simulink model "SDV_HIL"  (R2025a)
settings: Solver=VariableStepAuto  StartTime=0.0  StopTime=9999  FixedStep=0.001  RelTol=1e-3
undefined symbols (not defined in the file): Breakpoints_Fz, Cij, dspblkCoreblockFVToolHelper, eta, Fx_total_max, g, gcbh, Iz, lambda, lf, lr, mu, phi, R_eff, Tmax, xi
libraries: simulink_extras x30, slrealtimeiplib x17, slpidlib x16, simulink x10, SignalEditorBlockLib x6, dspstat3 x5, Solver_SF x3, sl3dlib x3
(part 4 of 5)

== system SDV_HIL/Draft1/UDP Transmit PC -> VCU1/Subsystem/Torque Vectoring/Speed Control ==
  Vx_des : Inport
  Vx : Inport  Port=2
  Display : Display  Commented=on
  MATLAB Function : MATLAB Function  TreatAsAtomicUnit=on
  Mux : Mux  Inputs=2
  PID Controller4 : slpidlib/PID Controller  Controller=PID  Form=Parallel  TimeDomain=Discrete-time  UseExternalTs=off  SampleTime=-1  IntegratorMethod=Forward Euler  FilterMethod=Forward Euler  ControllerParametersSource=internal  P=1500  I=2  UseKiTs=off  D=30  UseExternalDerivativeSource=off  N=100  UseFilter=on  TunerSelectOption=Transfer Function Based (PID Tuner App)  InitialConditionSource=internal  InitialConditionForIntegrator=0  InitialConditionForFilter=0  DifferentiatorICPrevScaledInput=0  ExternalReset=none  TrackingMode=off  Kt=1  LimitOutput=off  SatLimitsSource=internal  UpperSaturationLimit=inf  LowerSaturationLimit=-inf  LinearizeAsGain=on  AntiWindupMode=none  Kb=1  LimitIntegrator=off  UpperIntegratorSaturationLimit=inf  LowerIntegratorSaturationLimit=-inf  POutMin=[]  POutMax=[]  IOutMin=[]  IOutMax=[]  DOutMin=[]  DOutMax=[]  NOutMin=[]  NOutMax=[]  SumOutMin=[]  SumOutMax=[]  SaturationOutMin=[]  SaturationOutMax=[]  PParamMin=[]  PParamMax=[]  IParamMin=[]  IParamMax=[]  DParamMin=[]  DParamMax=[]  NParamMin=[]  NParamMax=[]  KbParamMin=[]  KbParamMax=[]  KtParamMin=[]  KtParamMax=[]  KbOutMin=[]  KbOutMax=[]  KtOutMin=[]  KtOutMax=[]  IntegratorOutMin=[]  IntegratorOutMax=[]  FilterOutMin=[]  FilterOutMax=[]  SumI1OutMin=[]  SumI1OutMax=[]  SumI2OutMin=[]  SumI2OutMax=[]  SumI3OutMin=[]  SumI3OutMax=[]  SumI4OutMin=[]  SumI4OutMax=[]  SumDOutMin=[]  SumDOutMax=[]  DifferentiatorOutMin=[]  DifferentiatorOutMax=[]  FilterDiffOutCoefMin=[]  FilterDiffOutCoefMax=[]  ReciprocalOutMin=[]  ReciprocalOutMax=[]  SumDenOutMin=[]  SumDenOutMax=[]  SumNumOutMin=[]  SumNumOutMax=[]  DivideOutMin=[]  DivideOutMax=[]  UdiffTsProdOutMin=[]  UdiffTsProdOutMax=[]  NTsProdOutMin=[]  NTsProdOutMax=[]  UintegralTsProdOutMin=[]  UintegralTsProdOutMax=[]  UngainTsProdOutMin=[]  UngainTsProdOutMax=[]  ClampingZeroOutDataTypeStr=Inherit: Inherit via back propagation  ClampingZeroOutMin=[]  ClampingZeroOutMax=[]  FilterDenConstantOutDataTypeStr=Inherit: Inherit via back propagation  FilterDenConstantOutMin=[]  FilterDenConstantOutMax=[]  PCopyOutDataTypeStr=Inherit: Inherit via back propagation  PCopyOutMin=[]  PCopyOutMax=[]  NCopyOutDataTypeStr=Inherit: Inherit via back propagation  NCopyOutMin=[]  NCopyOutMax=[]  IntegratorContinuousStateAttributes=''  IntegratorStateMustResolveToSignalObject=off  IntegratorRTWStateStorageClass=Auto  FilterContinuousStateAttributes=''  FilterStateMustResolveToSignalObject=off  FilterRTWStateStorageClass=Auto  ParallelPVariant=InternalParameters  IdealPVariant=Disabled  IVariant=InternalParameters  DVariant=InternalParameters  IntegratorVariant=Discrete  SatVariant=Disabled  AWVariant=Passthrough  PCopyVariant=Disabled  TRVariant=Disabled  FdbkBlocksVariant=Forward  IdealPFdbkVariant=Disabled  SatFdbkVariant=Disabled  DerivativeFilterVariant=ForwardEulerFilter  NVariant=InternalParameters  NCopyVariant=Disabled  FilterICVariant=InternalICsFilter  IntegratorICVariant=InternalICs  ExternalResetVariant=Disabled  TRSumVariant=Passthrough  SumFdbkVariant=Disabled  SumVariant=Sum_PID  TsampFilterVariant=InternalTs  TsampNgainVariant=Passthrough  TsampIntegralVariant=Disabled_SignalSpec  ExternalSaturationOutDataTypeStr=Inherit: Same as second input  DerivativeSourceVariant=ErrorSignal  PreIntVariant=InternalPreInt
  Saturation : Saturate  UpperLimit=Fx_total_max  LowerLimit=0
  Scope : Scope  Commented=on  NumInputPorts=2
      settings: ActiveDisplayYMinimum=-2.88760628149626  ActiveDisplayYMaximum=25.98790920244803  DataLoggingVariableName=ScopeData38
  Scope1 : Scope  Commented=on
      settings: ActiveDisplayYMinimum=-1  ActiveDisplayYMaximum=1  DataLoggingVariableName=ScopeData9
  Scope2 : Scope  Commented=on
      settings: DataLoggingVariableName=ScopeData64
  Sum1 : Sum  Inputs=|+-
  Fx_total : Outport
  tag scope: Vx_des=global
  wires:
  Vx_des/1 -> MATLAB Function/2(Vx_des), Mux/1, Sum1/1, [Vx_des]
  Vx/1 -> MATLAB Function/3(Vx), Mux/2, Sum1/2
  PID Controller4/1 -> Scope1/1, Saturation/1
  Mux/1 -> Scope/1
  Saturation/1 -> Scope/2, MATLAB Function/1(Fx_total)
  Sum1/1 -> PID Controller4/1
  MATLAB Function/1(y) -> Scope2/1, Display/1, Fx_total/1

== system SDV_HIL/Draft1/UDP Transmit PC -> VCU1/Subsystem/Torque Vectoring/Upper-Level Control ==
  r_des : Inport
  beta_des : Inport  Port=2
  r : Inport  Port=3
  beta : Inport  Port=4
  delta_in : Inport  Port=5
  Fy : Inport  Port=6
  Cos1 : Trigonometry  Operator=cos
  Demux : Demux  Outputs=2
  Demux1 : Demux
  Gain : Gain  Gain=lf
  Gain1 : Gain  Gain=lr
  Iz : Constant  Value=Iz
  Product : Product
  Product1 : Product
  Product2 : Product
  Reaching Law (sat) : Subsystem
  Scope{1..4} (4 alike) : Scope  Commented=on
      Scope1 settings: ActiveDisplayYMinimum=-17795.628494068122  ActiveDisplayYMaximum=19970.892039304985  DataLoggingVariableName=ScopeData_Mzd
      Scope2 settings: ActiveDisplayYMinimum=-0.48285830944080821  ActiveDisplayYMaximum=0.47895159374849061  DataLoggingVariableName=ScopeData_S
      Scope3 settings: DataLoggingVariableName=ScopeData_Sdot
      Scope4 settings: DataLoggingVariableName=ScopeData_rdotSmcMedfil
  Subtract : Sum  Inputs=+-+
  Sum1 : Sum  Inputs=|++
  Sum2 : Sum  Inputs=|++
  r_dot Calculation : Subsystem
      settings: PortSchema="{\"entries\":[{\"content\":{\"sides\":[{\"content\":{\"connectorIds\":[\"In1\",\"In2\",\"In3\"]},\"type\":\"ConnectorPlacement.EquallySpacedRectSide\",\"uuid\":\"24da7610-8c35-4174-a9dd-dc5523a7d40f\"},{\"content\":{\"connectorIds\":[\"Out1\"],\"side\":\"RIGHT\"},\"type\":\"ConnectorPlacement.EquallySpacedRectSide\",\"uuid\":\"8ddd6809-dcb9-493a-b194-91a4519159d8\"},{\"content\":{\"side\":\"TOP\"},\"type\":\"ConnectorPlacement.EquallySpacedRectSide\",\"uuid\":\"1e2c627d-8a14-4da0-8e59-ad29a76a798f\"},{\"content\":{\"connectorIds\":[\"In4\"],\"side\":\"BOTTOM\"},\"type\":\"ConnectorPlacement.EquallySpacedRectSide\",\"uuid\":\"4fc8884c-749f-4f20-8303-f46a5b29ae03\"}]},\"type\":\"ConnectorPlacement.EquallySpacedConnector\",\"uuid\":\"4c91258b-0c90-4974-b853-bf1095bd2674\"}],\"packageUris\":[\"http://schema.mathworks.com/mf0/Connector/R2020b\"],\"version\":\"1.0\"}"
  s Calculation : Subsystem
      settings: PortSchema="{\"entries\":[{\"content\":{\"sides\":[{\"content\":{\"connectorIds\":[\"In1\",\"In2\"]},\"type\":\"ConnectorPlacement.EquallySpacedRectSide\",\"uuid\":\"24da7610-8c35-4174-a9dd-dc5523a7d40f\"},{\"content\":{\"connectorIds\":[\"Out1\"],\"side\":\"RIGHT\"},\"type\":\"ConnectorPlacement.EquallySpacedRectSide\",\"uuid\":\"8ddd6809-dcb9-493a-b194-91a4519159d8\"},{\"content\":{\"side\":\"TOP\"},\"type\":\"ConnectorPlacement.EquallySpacedRectSide\",\"uuid\":\"1e2c627d-8a14-4da0-8e59-ad29a76a798f\"},{\"content\":{\"connectorIds\":[\"In3\",\"In4\"],\"side\":\"BOTTOM\"},\"type\":\"ConnectorPlacement.EquallySpacedRectSide\",\"uuid\":\"ef20af3e-2b8c-4d9e-a787-65384a3d573e\"}]},\"type\":\"ConnectorPlacement.EquallySpacedConnector\",\"uuid\":\"4c91258b-0c90-4974-b853-bf1095bd2674\"}],\"packageUris\":[\"http://schema.mathworks.com/mf0/Connector/R2020b\"],\"version\":\"1.0\"}"
  Mzd : Outport
  tag scope: beta_des=global
  wires:
  Sum1/1 -> Gain/1
  Sum2/1 -> Gain1/1
  Fy/1 -> Demux1/1
  s Calculation/1(s) -> Scope2/1, Reaching Law (sat)/1(s)  "s"
  Demux1/1 -> Sum1/1
  Subtract/1 -> Mzd/1, Scope1/1  "Mzd"
  Demux1/3 -> Sum2/1
  r_des/1 -> s Calculation/1(r_des), r_dot Calculation/1(r_des)
  Demux1/2 -> Sum1/2
  beta_des/1 -> [beta_des], s Calculation/2(beta_des), r_dot Calculation/2(beta_des)
  Product/1 -> Subtract/1
  Demux1/4 -> Sum2/2
  Iz/1 -> Product/2
  r_dot Calculation/1(r_dotSmc) -> Scope4/1, Product/1  "r_smc"
  Reaching Law (sat)/1(s_dot) -> Scope3/1, r_dot Calculation/3(s_dot)  "s_dot"
  r/1 -> s Calculation/3(r)
  beta/1 -> s Calculation/4(beta), r_dot Calculation/4(beta)
  Gain/1 -> Product1/1
  Product1/1 -> Subtract/2
  [wheelAng] -> Cos1/1
  Product2/1 -> Subtract/3
  Cos1/1 -> Demux/1
  Demux/1 -> Product1/2
  Demux/2 -> Product2/1
  Gain1/1 -> Product2/2
  delta_in/1 -> [wheelAng]

== system SDV_HIL/Draft1/UDP Transmit PC -> VCU1/Subsystem/Torque Vectoring/beta Calculations ==
  Vx : Inport
  Vy : Inport  Port=2
  Atan : Trigonometry  Operator=atan
  Constant1 : Constant  Value=1e-2
  Divide1 : Product  Inputs=*/
  Gain1 : Gain  Gain=1/3.6
  Gain2 : Gain  Gain=1/3.6
  Max : MinMax  Function=max  Inputs=2
  beta : Outport
  wires:
  Constant1/1 -> Max/1
  Atan/1 -> beta/1  "beta"
  Divide1/1 -> Atan/1
  Vx/1 -> Gain1/1
  Max/1 -> Divide1/2
  Gain2/1 -> Divide1/1
  Gain1/1 -> Max/2
  Vy/1 -> Gain2/1

== system SDV_HIL/Draft1/UDP Transmit PC -> VCU1/Subsystem/Torque Vectoring/delta_in Calculations ==
  AngWheel : Inport
  Add1 : Sum
  Add2 : Sum
  Constant : Constant  Value=2
  Constant1 : Constant  Value=2
  Demux1 : Demux
  Divide : Product  Inputs=*/
  Divide1 : Product  Inputs=*/
  Mux : Mux  Inputs=2
  delta_in : Outport
  wires:
  Constant/1 -> Divide/2
  Demux1/1 -> Add2/1
  Add2/1 -> Divide/1
  Demux1/2 -> Add2/2
  Demux1/4 -> Add1/2
  Demux1/3 -> Add1/1
  Add1/1 -> Divide1/1
  Constant1/1 -> Divide1/2
  Divide/1 -> Mux/1
  Divide1/1 -> Mux/2
  Mux/1 -> delta_in/1
  AngWheel/1 -> Demux1/1

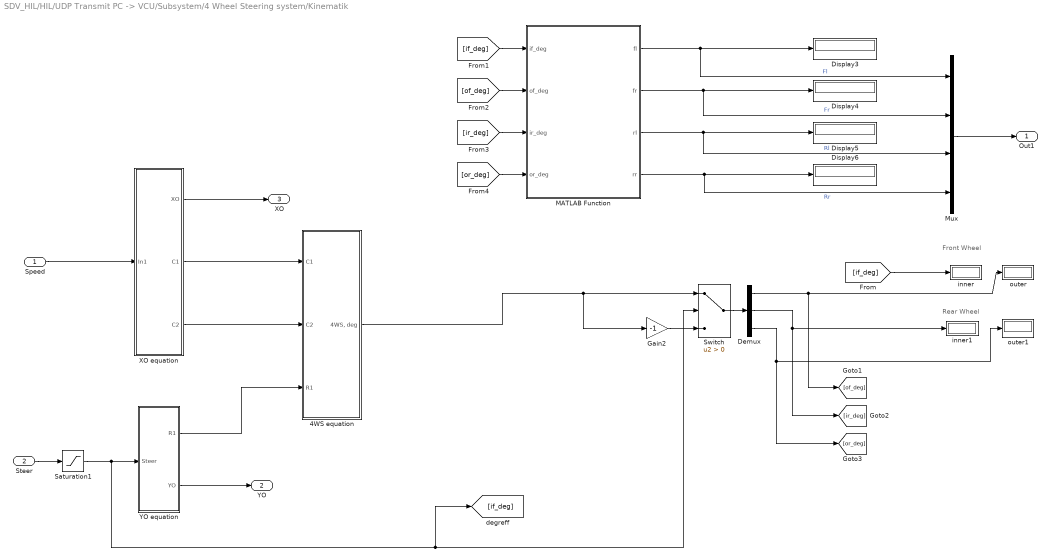
== system SDV_HIL/HIL/UDP Transmit PC -> VCU/Subsystem/4 Wheel Steering system/Kinematik ==
  note: Front Wheel
  note: Rear Wheel
  Speed : Inport
  Steer : Inport  Port=2
  4WS equation : Subsystem
  Demux : Demux  Outputs=3
  Display{3..6} (4 alike) : Display
  Gain2 : Gain  Gain=-1
  MATLAB Function : MATLAB Function  TreatAsAtomicUnit=on
  Mux : Mux
  Saturation1 : Saturate  UpperLimit=40  LowerLimit=-40
  Switch : Switch  Criteria=u2 > Threshold  SaturateOnIntegerOverflow=off  InputSameDT=off
  XO equation : Subsystem
  YO equation : Subsystem
  inner : Display
  inner1 : Display
  outer : Display
  outer1 : Display
  Out1 : Outport
  YO : Outport  Port=2
  XO : Outport  Port=3
  wires:
  Gain2/1 -> Switch/3
  Switch/1 -> Demux/1
  MATLAB Function/1(fl) -> Display3/1, Mux/1  "Fl"
  MATLAB Function/3(rl) -> Display5/1, Mux/3  "Rl"
  XO equation/1(XO) -> XO/1
  XO equation/2(C1) -> 4WS equation/1(C1)
  XO equation/3(C2) -> 4WS equation/2(C2)
  Steer/1 -> Saturation1/1
  YO equation/1(R1) -> 4WS equation/3(R1)
  YO equation/2(YO) -> YO/1
  4WS equation/1("4WS, deg") -> Gain2/1, Switch/1
  MATLAB Function/2(fr) -> Display4/1, Mux/2  "Fr"
  MATLAB Function/4(rr) -> Display6/1, Mux/4  "Rr"
  [if_deg] -> MATLAB Function/1(if_deg)
  [of_deg] -> MATLAB Function/2(of_deg)
  [ir_deg] -> MATLAB Function/3(ir_deg)
  [or_deg] -> MATLAB Function/4(or_deg)
  Demux/1 -> outer/1, [of_deg]
  Demux/3 -> outer1/1, [or_deg]
  Demux/2 -> inner1/1, [ir_deg]
  [if_deg] -> inner/1
  Mux/1 -> Out1/1
  Saturation1/1 -> [if_deg], Switch/2, YO equation/1(Steer)
  Speed/1 -> XO equation/1(In1)

== system SDV_HIL/HIL/UDP Transmit PC -> VCU/Subsystem/Torque Vectoring/Ca Calculations ==
  <Fz> : Inport
  1-D Lookup Table : Lookup_n-D  NumberOfTableDimensions=1  BreakpointsForDimension1=Breakpoints_Fz  Table=Cij  InternalRulePriority=Speed  RndMeth=Simplest
  Add : Sum
  Add1 : Sum
  Bus Creator2 : BusCreator  Inputs=2
  Demux : Demux
  Scope1 : Scope  Commented=on
      settings: ActiveDisplayYMinimum=151092.72809837208  ActiveDisplayYMaximum=177792.29609670336  DataLoggingVariableName=ScopeData_Cai
  Ca : Outport
  wires:
  Bus Creator2/1 -> Ca/1, Scope1/1  "Ca"
  Demux/1 -> Add/1  "FL"
  1-D Lookup Table/1 -> Demux/1
  Demux/2 -> Add/2  "FR"
  Demux/3 -> Add1/1  "RL"
  Add/1 -> Bus Creator2/1  "front"
  Demux/4 -> Add1/2  "RR"
  Add1/1 -> Bus Creator2/2  "rear"
  <Fz>/1 -> 1-D Lookup Table/1

== system SDV_HIL/HIL/UDP Transmit PC -> VCU/Subsystem/Torque Vectoring/Lower-Level Control ==
  Fx_total : Inport
  Mzd : Inport  Port=2
  delta_in : Inport  Port=3
  Fz : Inport  Port=4
  Constant : Constant  Value=4
  Constant1 : Constant  Value=mu
  Constant2 : Constant  Value=Tmax
  Display2 : Display  Commented=on
  Divide : Product  Inputs=*/
  Gain : Gain  Gain=R_eff
  Gain1 : Gain  Gain=4
  MATLAB Function1 : MATLAB Function  TreatAsAtomicUnit=on  SystemSampleTime=0.001
  Mux : Mux  Inputs=2
  Scope : Scope  Commented=on  NumInputPorts=2
      settings: ActiveDisplayYMinimum=-1280.000000001761  ActiveDisplayYMaximum=1280.0000000158495  DataLoggingVariableName=ScopeData44
  Scope1 : Scope  Commented=on  NumInputPorts=2
      settings: ActiveDisplayYMinimum=-9578.3971707250021  ActiveDisplayYMaximum=10211.837981002229  DataLoggingVariableName=ScopeData42
  Scope2 : Scope  Commented=on
      settings: ActiveDisplayYMinimum=-1.75  ActiveDisplayYMaximum=5.75  DataLoggingVariableName=ScopeData53
  Scope3 : Scope  Commented=on
      settings: ActiveDisplayYMinimum=-1  ActiveDisplayYMaximum=1  DataLoggingVariableName=ScopeData30
  Scope4 : Scope  Commented=on  NumInputPorts=3
      settings: ActiveDisplayYMinimum=-1734.1040462427745  ActiveDisplayYMaximum=1734.1040462427745  DataLoggingVariableName=ScopeData56
  Sum of Elements : Sum  Inputs=+
  Unit Delay : UnitDelay  InitialCondition=[0; 0; 0; 0]  SampleTime=-1  HasFrameUpgradeWarning=on
  TqMotorRef : Outport
  wires:
  Gain1/1 -> MATLAB Function1/5(Tshaft_max)
  Constant2/1 -> Gain1/1
  Mux/1 -> Scope3/1
  delta_in/1 -> MATLAB Function1/3(delta_in)
  Sum of Elements/1 -> Mux/2  "sum(Fx_opt)"
  Constant1/1 -> MATLAB Function1/6(mu)
  MATLAB Function1/3(Mx_total) -> Scope1/2  "Mx_total"
  Divide/1 -> TqMotorRef/1, Display2/1, Scope/2  "TqMotor"
  Constant/1 -> Divide/2
  MATLAB Function1/5(Fx_opt) -> Gain/1, Sum of Elements/1, Scope4/3, Unit Delay/1  "Fx_opt"
  Fz/1 -> MATLAB Function1/4(Fz)
  Mzd/1 -> Scope1/1, MATLAB Function1/2(Mzd)
  Fx_total/1 -> MATLAB Function1/1(Fx_total_ref), Mux/1
  Gain/1 -> Divide/1, Scope/1  "TqShaft"
  MATLAB Function1/4(exitflag) -> Scope2/1
  Unit Delay/1 -> MATLAB Function1/7(Fx_prev)
  MATLAB Function1/1(lb) -> Scope4/1  "lb"
  MATLAB Function1/2(ub) -> Scope4/2  "ub"

== system SDV_HIL/HIL/UDP Transmit PC -> VCU/Subsystem/Torque Vectoring/Reference Model ==
  delta_in : Inport
  Vx : Inport  Port=2
  Ca : Inport  Port=3
  Demux2 : Demux  Outputs=2
  Demux3 : Demux  Outputs=2
  Display : Display  Commented=on
  Draft : Subsystem  Commented=on
  Gain3 : Gain  Gain=-1
  Gain5 : Gain  Gain=-1
  Reference Model : MATLAB Function  TreatAsAtomicUnit=on
  Saturation Dynamic : simulink/Discontinuities/Saturation Dynamic  OutMin=[]  OutMax=[]  OutDataTypeStr=Inherit: Same as second input  OutDataType=fixdt(1, 16)  OutScaling=2^-10  DoSatur=off
  Saturation Dynamic1 : simulink/Discontinuities/Saturation Dynamic  OutMin=[]  OutMax=[]  OutDataTypeStr=Inherit: Same as second input  OutDataType=fixdt(1, 16)  OutScaling=2^-10  DoSatur=off
  Scope : Scope  Commented=on
      settings: ActiveDisplayYMinimum=-0.010237730942831622  ActiveDisplayYMaximum=0.0448211063407787  DataLoggingVariableName=ScopeData35
  Scope1 : Scope  Commented=on  NumInputPorts=2
      settings: ActiveDisplayYMinimum=-0.010237730942831622  ActiveDisplayYMaximum=0.0448211063407787  DataLoggingVariableName=ScopeData43
  Scope2 : Scope  Commented=on  NumInputPorts=2
      settings: ActiveDisplayYMinimum=-1  ActiveDisplayYMaximum=1  DataLoggingVariableName=ScopeData45
  Scope3 : Scope  Commented=on  NumInputPorts=2
      settings: ActiveDisplayYMinimum=-0.28358581685431428  ActiveDisplayYMaximum=0.28405537038366757  DataLoggingVariableName=ScopeData41
  Selector : Selector  InputPortWidth=2  IndexOptions=Index vector (dialog)  Indices=[1]  OutputSizes=1
  r&beta Limiter : Subsystem
  r_des : Outport
  beta_des : Outport  Port=2
  wires:
  Demux3/1 -> Scope1/1, Saturation Dynamic/2  "r_des"
  Demux2/1 -> Reference Model/3(Caf)
  Demux2/2 -> Reference Model/4(Car)
  Vx/1 -> r&beta Limiter/1(Vx), Reference Model/2(Vx)
  Demux3/2 -> Scope2/1, Saturation Dynamic1/2  "beta_des"
  delta_in/1 -> Selector/1
  Ca/1 -> Demux2/1
  Reference Model/1(y) -> Scope/1, Demux3/1  "r & beta_des"
  Gain3/1 -> Saturation Dynamic/3
  Saturation Dynamic/1 -> Display/1, r_des/1, Scope3/1, Scope1/2  "r_desUnsat"
  Gain5/1 -> Saturation Dynamic1/3
  Saturation Dynamic1/1 -> Scope2/2, beta_des/1, Scope3/2  "beta_desUnsat"
  r&beta Limiter/1(rLim) -> Gain3/1, Saturation Dynamic/1
  r&beta Limiter/2(betaLim) -> Saturation Dynamic1/1, Gain5/1
  Selector/1 -> Reference Model/1(delta_in)

== system SDV_HIL/HIL/UDP Transmit PC -> VCU/Subsystem/Torque Vectoring/Speed Control ==
  Vx_des : Inport
  Vx : Inport  Port=2
  Display : Display  Commented=on
  MATLAB Function : MATLAB Function  TreatAsAtomicUnit=on
  Mux : Mux  Inputs=2
  PID Controller4 : slpidlib/PID Controller  Controller=PID  Form=Parallel  TimeDomain=Discrete-time  UseExternalTs=off  SampleTime=-1  IntegratorMethod=Forward Euler  FilterMethod=Forward Euler  ControllerParametersSource=internal  P=1500  I=2  UseKiTs=off  D=30  UseExternalDerivativeSource=off  N=100  UseFilter=on  TunerSelectOption=Transfer Function Based (PID Tuner App)  InitialConditionSource=internal  InitialConditionForIntegrator=0  InitialConditionForFilter=0  DifferentiatorICPrevScaledInput=0  ExternalReset=none  TrackingMode=off  Kt=1  LimitOutput=off  SatLimitsSource=internal  UpperSaturationLimit=inf  LowerSaturationLimit=-inf  LinearizeAsGain=on  AntiWindupMode=none  Kb=1  LimitIntegrator=off  UpperIntegratorSaturationLimit=inf  LowerIntegratorSaturationLimit=-inf  POutMin=[]  POutMax=[]  IOutMin=[]  IOutMax=[]  DOutMin=[]  DOutMax=[]  NOutMin=[]  NOutMax=[]  SumOutMin=[]  SumOutMax=[]  SaturationOutMin=[]  SaturationOutMax=[]  PParamMin=[]  PParamMax=[]  IParamMin=[]  IParamMax=[]  DParamMin=[]  DParamMax=[]  NParamMin=[]  NParamMax=[]  KbParamMin=[]  KbParamMax=[]  KtParamMin=[]  KtParamMax=[]  KbOutMin=[]  KbOutMax=[]  KtOutMin=[]  KtOutMax=[]  IntegratorOutMin=[]  IntegratorOutMax=[]  FilterOutMin=[]  FilterOutMax=[]  SumI1OutMin=[]  SumI1OutMax=[]  SumI2OutMin=[]  SumI2OutMax=[]  SumI3OutMin=[]  SumI3OutMax=[]  SumI4OutMin=[]  SumI4OutMax=[]  SumDOutMin=[]  SumDOutMax=[]  DifferentiatorOutMin=[]  DifferentiatorOutMax=[]  FilterDiffOutCoefMin=[]  FilterDiffOutCoefMax=[]  ReciprocalOutMin=[]  ReciprocalOutMax=[]  SumDenOutMin=[]  SumDenOutMax=[]  SumNumOutMin=[]  SumNumOutMax=[]  DivideOutMin=[]  DivideOutMax=[]  UdiffTsProdOutMin=[]  UdiffTsProdOutMax=[]  NTsProdOutMin=[]  NTsProdOutMax=[]  UintegralTsProdOutMin=[]  UintegralTsProdOutMax=[]  UngainTsProdOutMin=[]  UngainTsProdOutMax=[]  ClampingZeroOutDataTypeStr=Inherit: Inherit via back propagation  ClampingZeroOutMin=[]  ClampingZeroOutMax=[]  FilterDenConstantOutDataTypeStr=Inherit: Inherit via back propagation  FilterDenConstantOutMin=[]  FilterDenConstantOutMax=[]  PCopyOutDataTypeStr=Inherit: Inherit via back propagation  PCopyOutMin=[]  PCopyOutMax=[]  NCopyOutDataTypeStr=Inherit: Inherit via back propagation  NCopyOutMin=[]  NCopyOutMax=[]  IntegratorContinuousStateAttributes=''  IntegratorStateMustResolveToSignalObject=off  IntegratorRTWStateStorageClass=Auto  FilterContinuousStateAttributes=''  FilterStateMustResolveToSignalObject=off  FilterRTWStateStorageClass=Auto  ParallelPVariant=InternalParameters  IdealPVariant=Disabled  IVariant=InternalParameters  DVariant=InternalParameters  IntegratorVariant=Discrete  SatVariant=Disabled  AWVariant=Passthrough  PCopyVariant=Disabled  TRVariant=Disabled  FdbkBlocksVariant=Forward  IdealPFdbkVariant=Disabled  SatFdbkVariant=Disabled  DerivativeFilterVariant=ForwardEulerFilter  NVariant=InternalParameters  NCopyVariant=Disabled  FilterICVariant=InternalICsFilter  IntegratorICVariant=InternalICs  ExternalResetVariant=Disabled  TRSumVariant=Passthrough  SumFdbkVariant=Disabled  SumVariant=Sum_PID  TsampFilterVariant=InternalTs  TsampNgainVariant=Passthrough  TsampIntegralVariant=Disabled_SignalSpec  ExternalSaturationOutDataTypeStr=Inherit: Same as second input  DerivativeSourceVariant=ErrorSignal  PreIntVariant=InternalPreInt
  Saturation : Saturate  UpperLimit=Fx_total_max  LowerLimit=0
  Scope : Scope  Commented=on  NumInputPorts=2
      settings: ActiveDisplayYMinimum=-2.88760628149626  ActiveDisplayYMaximum=25.98790920244803  DataLoggingVariableName=ScopeData38
  Scope1 : Scope  Commented=on
      settings: ActiveDisplayYMinimum=-1  ActiveDisplayYMaximum=1  DataLoggingVariableName=ScopeData9
  Scope2 : Scope  Commented=on
      settings: DataLoggingVariableName=ScopeData64
  Sum1 : Sum  Inputs=|+-
  Fx_total : Outport
  tag scope: Vx_des=global
  wires:
  Vx_des/1 -> MATLAB Function/2(Vx_des), Mux/1, Sum1/1, [Vx_des]
  Vx/1 -> MATLAB Function/3(Vx), Mux/2, Sum1/2
  PID Controller4/1 -> Scope1/1, Saturation/1
  Mux/1 -> Scope/1
  Saturation/1 -> Scope/2, MATLAB Function/1(Fx_total)
  Sum1/1 -> PID Controller4/1
  MATLAB Function/1(y) -> Scope2/1, Display/1, Fx_total/1

== system SDV_HIL/HIL/UDP Transmit PC -> VCU/Subsystem/Torque Vectoring/Upper-Level Control ==
  r_des : Inport
  beta_des : Inport  Port=2
  r : Inport  Port=3
  beta : Inport  Port=4
  delta_in : Inport  Port=5
  Fy : Inport  Port=6
  Cos1 : Trigonometry  Operator=cos
  Demux : Demux  Outputs=2
  Demux1 : Demux
  Gain : Gain  Gain=lf
  Gain1 : Gain  Gain=lr
  Iz : Constant  Value=Iz
  Product : Product
  Product1 : Product
  Product2 : Product
  Reaching Law (sat) : Subsystem
  Scope{1..4} (4 alike) : Scope  Commented=on
      Scope1 settings: ActiveDisplayYMinimum=-17795.628494068122  ActiveDisplayYMaximum=19970.892039304985  DataLoggingVariableName=ScopeData_Mzd
      Scope2 settings: ActiveDisplayYMinimum=-0.48285830944080821  ActiveDisplayYMaximum=0.47895159374849061  DataLoggingVariableName=ScopeData_S
      Scope3 settings: DataLoggingVariableName=ScopeData_Sdot
      Scope4 settings: DataLoggingVariableName=ScopeData_rdotSmcMedfil
  Subtract : Sum  Inputs=+-+
  Sum1 : Sum  Inputs=|++
  Sum2 : Sum  Inputs=|++
  r_dot Calculation : Subsystem
      settings: PortSchema="{\"entries\":[{\"content\":{\"sides\":[{\"content\":{\"connectorIds\":[\"In1\",\"In2\",\"In3\"]},\"type\":\"ConnectorPlacement.EquallySpacedRectSide\",\"uuid\":\"24da7610-8c35-4174-a9dd-dc5523a7d40f\"},{\"content\":{\"connectorIds\":[\"Out1\"],\"side\":\"RIGHT\"},\"type\":\"ConnectorPlacement.EquallySpacedRectSide\",\"uuid\":\"8ddd6809-dcb9-493a-b194-91a4519159d8\"},{\"content\":{\"side\":\"TOP\"},\"type\":\"ConnectorPlacement.EquallySpacedRectSide\",\"uuid\":\"1e2c627d-8a14-4da0-8e59-ad29a76a798f\"},{\"content\":{\"connectorIds\":[\"In4\"],\"side\":\"BOTTOM\"},\"type\":\"ConnectorPlacement.EquallySpacedRectSide\",\"uuid\":\"4fc8884c-749f-4f20-8303-f46a5b29ae03\"}]},\"type\":\"ConnectorPlacement.EquallySpacedConnector\",\"uuid\":\"4c91258b-0c90-4974-b853-bf1095bd2674\"}],\"packageUris\":[\"http://schema.mathworks.com/mf0/Connector/R2020b\"],\"version\":\"1.0\"}"
  s Calculation : Subsystem
      settings: PortSchema="{\"entries\":[{\"content\":{\"sides\":[{\"content\":{\"connectorIds\":[\"In1\",\"In2\"]},\"type\":\"ConnectorPlacement.EquallySpacedRectSide\",\"uuid\":\"24da7610-8c35-4174-a9dd-dc5523a7d40f\"},{\"content\":{\"connectorIds\":[\"Out1\"],\"side\":\"RIGHT\"},\"type\":\"ConnectorPlacement.EquallySpacedRectSide\",\"uuid\":\"8ddd6809-dcb9-493a-b194-91a4519159d8\"},{\"content\":{\"side\":\"TOP\"},\"type\":\"ConnectorPlacement.EquallySpacedRectSide\",\"uuid\":\"1e2c627d-8a14-4da0-8e59-ad29a76a798f\"},{\"content\":{\"connectorIds\":[\"In3\",\"In4\"],\"side\":\"BOTTOM\"},\"type\":\"ConnectorPlacement.EquallySpacedRectSide\",\"uuid\":\"ef20af3e-2b8c-4d9e-a787-65384a3d573e\"}]},\"type\":\"ConnectorPlacement.EquallySpacedConnector\",\"uuid\":\"4c91258b-0c90-4974-b853-bf1095bd2674\"}],\"packageUris\":[\"http://schema.mathworks.com/mf0/Connector/R2020b\"],\"version\":\"1.0\"}"
  Mzd : Outport
  tag scope: Mzd=global, beta_des=global
  wires:
  Sum1/1 -> Gain/1
  Sum2/1 -> Gain1/1
  Fy/1 -> Demux1/1
  s Calculation/1(s) -> Scope2/1, Reaching Law (sat)/1(s)  "s"
  Demux1/1 -> Sum1/1
  Subtract/1 -> [Mzd], Mzd/1, Scope1/1  "Mzd"
  Demux1/3 -> Sum2/1
  r_des/1 -> s Calculation/1(r_des), r_dot Calculation/1(r_des)
  Demux1/2 -> Sum1/2
  beta_des/1 -> [beta_des], s Calculation/2(beta_des), r_dot Calculation/2(beta_des)
  Product/1 -> Subtract/1
  Demux1/4 -> Sum2/2
  Iz/1 -> Product/2
  r_dot Calculation/1(r_dotSmc) -> Scope4/1, Product/1  "r_smc"
  Reaching Law (sat)/1(s_dot) -> Scope3/1, r_dot Calculation/3(s_dot)  "s_dot"
  r/1 -> s Calculation/3(r)
  beta/1 -> s Calculation/4(beta), r_dot Calculation/4(beta)
  Gain/1 -> Product1/1
  Product1/1 -> Subtract/2
  [wheelAng] -> Cos1/1
  Product2/1 -> Subtract/3
  Cos1/1 -> Demux/1
  Demux/1 -> Product1/2
  Demux/2 -> Product2/1
  Gain1/1 -> Product2/2
  delta_in/1 -> [wheelAng]

== system SDV_HIL/HIL/UDP Transmit PC -> VCU/Subsystem/Torque Vectoring/beta Calculations ==
  Vx : Inport
  Vy : Inport  Port=2
  Atan : Trigonometry  Operator=atan
  Constant1 : Constant  Value=1e-2
  Divide1 : Product  Inputs=*/
  Gain1 : Gain  Gain=1/3.6
  Gain2 : Gain  Gain=1/3.6
  Max : MinMax  Function=max  Inputs=2
  beta : Outport
  wires:
  Constant1/1 -> Max/1
  Atan/1 -> beta/1  "beta"
  Divide1/1 -> Atan/1
  Vx/1 -> Gain1/1
  Max/1 -> Divide1/2
  Gain2/1 -> Divide1/1
  Gain1/1 -> Max/2
  Vy/1 -> Gain2/1

== system SDV_HIL/HIL/UDP Transmit PC -> VCU/Subsystem/Torque Vectoring/delta_in Calculations ==
  AngWheel : Inport
  Add1 : Sum
  Add2 : Sum
  Constant : Constant  Value=2
  Constant1 : Constant  Value=2
  Demux1 : Demux
  Divide : Product  Inputs=*/
  Divide1 : Product  Inputs=*/
  Mux : Mux  Inputs=2
  delta_in : Outport
  wires:
  Constant/1 -> Divide/2
  Demux1/1 -> Add2/1
  Add2/1 -> Divide/1
  Demux1/2 -> Add2/2
  Demux1/4 -> Add1/2
  Demux1/3 -> Add1/1
  Add1/1 -> Divide1/1
  Constant1/1 -> Divide1/2
  Divide/1 -> Mux/1
  Divide1/1 -> Mux/2
  Mux/1 -> delta_in/1
  AngWheel/1 -> Demux1/1

== system SDV_HIL/Draft1/UDP Transmit PC -> VCU1/Subsystem/4 Wheel Steering system/Kinematik/4WS equation ==
  C1 : Inport
  C2 : Inport  Port=2
  R1 : Inport  Port=3
  MATLAB Function : MATLAB Function  TreatAsAtomicUnit=on
  Mux : Mux  Inputs=3
  "4WS, deg" : Outport
  wires:
  Mux/1 -> "4WS, deg"/1
  MATLAB Function/1(of) -> Mux/1
  MATLAB Function/2(ir) -> Mux/2
  C1/1 -> MATLAB Function/1(C1)
  C2/1 -> MATLAB Function/2(C2)
  R1/1 -> MATLAB Function/3(R1)
  MATLAB Function/3(or) -> Mux/3

== system SDV_HIL/Draft1/UDP Transmit PC -> VCU1/Subsystem/4 Wheel Steering system/Kinematik/XO equation ==
  In1 : Inport
  1-D Lookup Table : Lookup_n-D  NumberOfTableDimensions=1  BreakpointsForDimension1=[0, 10, 20, 30, 40, 50, 55, 60]  Table=[1.55,1.86,2.165,2.47,2.78,3.1,3.4775,3.855]  InternalRulePriority=Speed  RndMeth=Simplest
  Constant : Constant  Value=1.55
  MATLAB Function : MATLAB Function  TreatAsAtomicUnit=on
  Saturation2 : Saturate  UpperLimit=3.855  LowerLimit=1.55
  XO : Outport
  C1 : Outport  Port=2
  C2 : Outport  Port=3
  wires:
  Constant/1 -> C1/1
  MATLAB Function/2(C2) -> C2/1
  MATLAB Function/1(X0) -> XO/1
  1-D Lookup Table/1 -> Saturation2/1
  Saturation2/1 -> MATLAB Function/1(Speed)
  In1/1 -> 1-D Lookup Table/1

== system SDV_HIL/Draft1/UDP Transmit PC -> VCU1/Subsystem/4 Wheel Steering system/Kinematik/YO equation ==
  Steer : Inport
  MATLAB Function : MATLAB Function  TreatAsAtomicUnit=on
  Subsystem : Subsystem  Commented=on
  R1 : Outport
  YO : Outport  Port=2
  wires:
  Steer/1 -> MATLAB Function/1(Steer)
  MATLAB Function/2(Y0) -> YO/1
  MATLAB Function/1(R1) -> R1/1

== system SDV_HIL/Draft1/UDP Transmit PC -> VCU1/Subsystem/Torque Vectoring/Reference Model/Draft ==
  MATLAB Function1 : MATLAB Function  TreatAsAtomicUnit=on
  MATLAB Function2 : MATLAB Function  TreatAsAtomicUnit=on

== system SDV_HIL/Draft1/UDP Transmit PC -> VCU1/Subsystem/Torque Vectoring/Reference Model/r&beta Limiter ==
  Vx : Inport
  Atan : Trigonometry  Operator=atan
  Constant : Constant  Value=1e-2
  Divide : Product  Inputs=*/
  Gain : Gain  Gain=g
  Gain1 : Gain  Gain=1/3.6
  Gain2 : Gain  Gain=0.85
  Gain4 : Gain  Gain=0.02
  Max : MinMax  Function=max  Inputs=2
  mu : Constant  Value=mu
  rLim : Outport
  betaLim : Outport  Port=2
  wires:
  Gain4/1 -> Atan/1
  Gain2/1 -> rLim/1
  Divide/1 -> Gain2/1
  Gain/1 -> Divide/1, Gain4/1
  mu/1 -> Gain/1
  Vx/1 -> Gain1/1
  Atan/1 -> betaLim/1
  Gain1/1 -> Max/1  "km/h -> m/s"
  Constant/1 -> Max/2
  Max/1 -> Divide/2

== system SDV_HIL/Draft1/UDP Transmit PC -> VCU1/Subsystem/Torque Vectoring/Upper-Level Control/Reaching Law (sat) ==
  note: saturation
  s : Inport
  Divide : Product  Inputs=*/
  Phi : Constant  Value=phi
  Saturation : Saturate  UpperLimit=1  LowerLimit=-1
  Scope : Scope  Commented=on
      settings: ActiveDisplayYMinimum=-1  ActiveDisplayYMaximum=1  DataLoggingVariableName=ScopeData40
  Scope1 : Scope  Commented=on
      settings: ActiveDisplayYMinimum=-1  ActiveDisplayYMaximum=1
  Scope2 : Scope  Commented=on  NumInputPorts=2
      settings: ActiveDisplayYMinimum=-0.20132018708021746  ActiveDisplayYMaximum=0.1978540927182815  DataLoggingVariableName=ScopeData47
  Subtract : Sum  Inputs=--
  eta : Gain  Gain=eta
  lambda : Gain  Gain=lambda
  s_dot : Outport
  wires:
  Divide/1 -> Saturation/1
  lambda/1 -> Scope/1, Subtract/2
  eta/1 -> Scope1/1, Subtract/1
  Subtract/1 -> Scope2/2, s_dot/1  "s_dot"
  Phi/1 -> Divide/2
  s/1 -> Divide/1, Scope2/1, eta/1
  Saturation/1 -> lambda/1

== system SDV_HIL/Draft1/UDP Transmit PC -> VCU1/Subsystem/Torque Vectoring/Upper-Level Control/r_dot Calculation ==
  r_des : Inport
  beta_des : Inport  Port=2
  s_dot : Inport  Port=3
  beta : Inport  Port=4
  Discrete Derivative : simulink/Discrete/Discrete Derivative  gainval=1.0  ICPrevScaledInput=0.0  OutMin=[]  OutMax=[]  OutDataType=fixdt(1, 16)  OutScaling=2^-10  DoSatur=off
  Discrete Derivative1 : simulink/Discrete/Discrete Derivative  gainval=1.0  ICPrevScaledInput=0.0  OutMin=[]  OutMax=[]  OutDataType=fixdt(1, 16)  OutScaling=2^-10  DoSatur=off
  Discrete Derivative2 : simulink/Discrete/Discrete Derivative  gainval=1.0  ICPrevScaledInput=0.0  OutMin=[]  OutMax=[]  OutDataType=fixdt(1, 16)  OutScaling=2^-10  DoSatur=off
  Draft : Subsystem  Commented=on
  Median Filter : dspstat3/Median Filter  WindowLength=3  SimulateUsing=Interpreted execution
      settings: LibrarySourceBlock=|
      | dspfdesign/Median
      | Filter
  Scope : Scope  Commented=on
      settings: ActiveDisplayYMinimum=-1  ActiveDisplayYMaximum=1  DataLoggingVariableName=ScopeData54
  Scope1 : Scope  Commented=on  NumInputPorts=2
      settings: ActiveDisplayYMinimum=-32.042890877269073  ActiveDisplayYMaximum=34.967572489026168  DataLoggingVariableName=ScopeData48
  Scope2 : Scope  Commented=on
      settings: ActiveDisplayYMinimum=-1.959672445143287  ActiveDisplayYMaximum=1.8206301349989764  DataLoggingVariableName=ScopeData55
  Scope3 : Scope  Commented=on  NumInputPorts=2
      settings: ActiveDisplayYMinimum=-4.3284275921621367  ActiveDisplayYMaximum=4.2312214706255107  DataLoggingVariableName=ScopeData50
  Scope4 : Scope  Commented=on
      settings: DataLoggingVariableName=ScopeData_rdotSmc
  Subtract : Sum  Inputs=+-
  Sum3 : Sum  Inputs=|++
  Sum4 : Sum  Inputs=|+-
  xi1 : Gain  Gain=xi
  r_dotSmc : Outport
  tag scope: r_dotSmc=global
  wires:
  Sum4/1 -> xi1/1
  xi1/1 -> Scope1/2, Subtract/2
  Discrete Derivative1/1 -> Sum4/1
  Sum3/1 -> Scope1/1, Subtract/1
  Discrete Derivative/1 -> Sum3/2
  s_dot/1 -> Sum3/1
  Discrete Derivative2/1 -> Sum4/2
  Subtract/1 -> Scope4/1, [r_dotSmc], Scope3/1, Scope2/1, Median Filter/1  "r_dotSmc"
  Median Filter/1 -> r_dotSmc/1, Scope/1, Scope3/2  "r_dotSmc"
  r_des/1 -> Discrete Derivative/1
  beta/1 -> Discrete Derivative1/1
  beta_des/1 -> Discrete Derivative2/1

== system SDV_HIL/Draft1/UDP Transmit PC -> VCU1/Subsystem/Torque Vectoring/Upper-Level Control/s Calculation ==
  r_des : Inport
  beta_des : Inport  Port=2
  r : Inport  Port=3
  beta : Inport  Port=4
  Add : Sum
  Mux : Mux  Inputs=2
  Mux1 : Mux  Inputs=2
  Mux2 : Mux  Inputs=2
  Radians to Degrees : simulink_extras/Transformations/Radians to Degrees
  Radians to Degrees1 : simulink_extras/Transformations/Radians to Degrees
  Scope : Scope  Commented=on  NumInputPorts=2
      settings: ActiveDisplayYMinimum=-0.28171028288036076  ActiveDisplayYMaximum=0.28186498160357804  DataLoggingVariableName=ScopeData27
  Scope1 : Scope  Commented=on  NumInputPorts=2
      settings: ActiveDisplayYMinimum=-0.14632790991396921  ActiveDisplayYMaximum=0.14632790991396921  DataLoggingVariableName=ScopeData28
  Scope2 : Scope  Commented=on
      settings: ActiveDisplayYMinimum=-15.502678068808111  ActiveDisplayYMaximum=19.821343432137777  DataLoggingVariableName=ScopeData_rRespons
  Scope3 : Scope  Commented=on
      settings: ActiveDisplayYMinimum=-5.2852193383146249  ActiveDisplayYMaximum=3.969293753648568  DataLoggingVariableName=ScopeData_betaRespons
  Sum1 : Sum  Inputs=|+-
  Sum2 : Sum  Inputs=|+-
  xi : Gain  Gain=xi
  s : Outport
  tag scope: rBeta_respons=global
  wires:
  Add/1 -> s/1
  xi/1 -> Add/2
  Sum2/1 -> xi/1  "err_beta"
  Sum1/1 -> Add/1  "error_yawrate"
  r/1 -> Mux/2, Scope/2, Sum1/1
  r_des/1 -> Mux/1, Scope/1, Sum1/2
  beta/1 -> Mux1/2, Scope1/2, Sum2/1
  Mux/1 -> Mux2/1, Radians to Degrees/1
  Mux1/1 -> Mux2/2, Radians to Degrees1/1
  Mux2/1 -> [rBeta_respons]
  Radians to Degrees/1 -> Scope2/1
  Radians to Degrees1/1 -> Scope3/1
  beta_des/1 -> Mux1/1, Scope1/1, Sum2/2

== system SDV_HIL/HIL/UDP Transmit PC -> VCU/Subsystem/4 Wheel Steering system/Kinematik/4WS equation ==
  C1 : Inport
  C2 : Inport  Port=2
  R1 : Inport  Port=3
  MATLAB Function : MATLAB Function  TreatAsAtomicUnit=on
  Mux : Mux  Inputs=3
  "4WS, deg" : Outport
  wires:
  Mux/1 -> "4WS, deg"/1
  MATLAB Function/1(of) -> Mux/1
  MATLAB Function/2(ir) -> Mux/2
  C1/1 -> MATLAB Function/1(C1)
  C2/1 -> MATLAB Function/2(C2)
  R1/1 -> MATLAB Function/3(R1)
  MATLAB Function/3(or) -> Mux/3

== system SDV_HIL/HIL/UDP Transmit PC -> VCU/Subsystem/4 Wheel Steering system/Kinematik/XO equation ==
  In1 : Inport
  1-D Lookup Table : Lookup_n-D  NumberOfTableDimensions=1  BreakpointsForDimension1=[0, 10, 20, 30, 40, 50, 55, 60]  Table=[1.55,1.86,2.165,2.47,2.78,3.1,3.4775,3.855]  InternalRulePriority=Speed  RndMeth=Simplest
  Constant : Constant  Value=1.55
  MATLAB Function : MATLAB Function  TreatAsAtomicUnit=on
  Saturation2 : Saturate  UpperLimit=3.855  LowerLimit=1.55
  XO : Outport
  C1 : Outport  Port=2
  C2 : Outport  Port=3
  wires:
  Constant/1 -> C1/1
  MATLAB Function/2(C2) -> C2/1
  MATLAB Function/1(X0) -> XO/1
  1-D Lookup Table/1 -> Saturation2/1
  Saturation2/1 -> MATLAB Function/1(Speed)
  In1/1 -> 1-D Lookup Table/1

== system SDV_HIL/HIL/UDP Transmit PC -> VCU/Subsystem/4 Wheel Steering system/Kinematik/YO equation ==
  Steer : Inport
  MATLAB Function : MATLAB Function  TreatAsAtomicUnit=on
  Subsystem : Subsystem  Commented=on
  R1 : Outport
  YO : Outport  Port=2
  wires:
  Steer/1 -> MATLAB Function/1(Steer)
  MATLAB Function/2(Y0) -> YO/1
  MATLAB Function/1(R1) -> R1/1

== system SDV_HIL/HIL/UDP Transmit PC -> VCU/Subsystem/Torque Vectoring/Reference Model/Draft ==
  MATLAB Function1 : MATLAB Function  TreatAsAtomicUnit=on
  MATLAB Function2 : MATLAB Function  TreatAsAtomicUnit=on

== system SDV_HIL/HIL/UDP Transmit PC -> VCU/Subsystem/Torque Vectoring/Reference Model/r&beta Limiter ==
  Vx : Inport
  Atan : Trigonometry  Operator=atan
  Constant : Constant  Value=1e-2
  Divide : Product  Inputs=*/
  Gain : Gain  Gain=g
  Gain1 : Gain  Gain=1/3.6
  Gain2 : Gain  Gain=0.85
  Gain4 : Gain  Gain=0.02
  Max : MinMax  Function=max  Inputs=2
  mu : Constant  Value=mu
  rLim : Outport
  betaLim : Outport  Port=2
  wires:
  Gain4/1 -> Atan/1
  Gain2/1 -> rLim/1
  Divide/1 -> Gain2/1
  Gain/1 -> Divide/1, Gain4/1
  mu/1 -> Gain/1
  Vx/1 -> Gain1/1
  Atan/1 -> betaLim/1
  Gain1/1 -> Max/1  "km/h -> m/s"
  Constant/1 -> Max/2
  Max/1 -> Divide/2

== system SDV_HIL/HIL/UDP Transmit PC -> VCU/Subsystem/Torque Vectoring/Upper-Level Control/Reaching Law (sat) ==
  note: saturation
  s : Inport
  Divide : Product  Inputs=*/
  Phi : Constant  Value=phi
  Saturation : Saturate  UpperLimit=1  LowerLimit=-1
  Scope : Scope  Commented=on
      settings: ActiveDisplayYMinimum=-1  ActiveDisplayYMaximum=1  DataLoggingVariableName=ScopeData40
  Scope1 : Scope  Commented=on
      settings: ActiveDisplayYMinimum=-1  ActiveDisplayYMaximum=1
  Scope2 : Scope  Commented=on  NumInputPorts=2
      settings: ActiveDisplayYMinimum=-0.20132018708021746  ActiveDisplayYMaximum=0.1978540927182815  DataLoggingVariableName=ScopeData47
  Subtract : Sum  Inputs=--
  eta : Gain  Gain=eta
  lambda : Gain  Gain=lambda
  s_dot : Outport
  wires:
  Divide/1 -> Saturation/1
  lambda/1 -> Scope/1, Subtract/2
  eta/1 -> Scope1/1, Subtract/1
  Subtract/1 -> Scope2/2, s_dot/1  "s_dot"
  Phi/1 -> Divide/2
  s/1 -> Divide/1, Scope2/1, eta/1
  Saturation/1 -> lambda/1

== system SDV_HIL/HIL/UDP Transmit PC -> VCU/Subsystem/Torque Vectoring/Upper-Level Control/r_dot Calculation ==
  r_des : Inport
  beta_des : Inport  Port=2
  s_dot : Inport  Port=3
  beta : Inport  Port=4
  Discrete Derivative : simulink/Discrete/Discrete Derivative  gainval=1.0  ICPrevScaledInput=0.0  OutMin=[]  OutMax=[]  OutDataType=fixdt(1, 16)  OutScaling=2^-10  DoSatur=off
  Discrete Derivative1 : simulink/Discrete/Discrete Derivative  gainval=1.0  ICPrevScaledInput=0.0  OutMin=[]  OutMax=[]  OutDataType=fixdt(1, 16)  OutScaling=2^-10  DoSatur=off
  Discrete Derivative2 : simulink/Discrete/Discrete Derivative  gainval=1.0  ICPrevScaledInput=0.0  OutMin=[]  OutMax=[]  OutDataType=fixdt(1, 16)  OutScaling=2^-10  DoSatur=off
  Draft : Subsystem  Commented=on
  Median Filter : dspstat3/Median Filter  WindowLength=3  SimulateUsing=Interpreted execution
      settings: LibrarySourceBlock=|
      | dspfdesign/Median
      | Filter
  Scope : Scope  Commented=on
      settings: ActiveDisplayYMinimum=-1  ActiveDisplayYMaximum=1  DataLoggingVariableName=ScopeData54
  Scope1 : Scope  Commented=on  NumInputPorts=2
      settings: ActiveDisplayYMinimum=-32.042890877269073  ActiveDisplayYMaximum=34.967572489026168  DataLoggingVariableName=ScopeData48
  Scope2 : Scope  Commented=on
      settings: ActiveDisplayYMinimum=-1.959672445143287  ActiveDisplayYMaximum=1.8206301349989764  DataLoggingVariableName=ScopeData55
  Scope3 : Scope  Commented=on  NumInputPorts=2
      settings: ActiveDisplayYMinimum=-4.3284275921621367  ActiveDisplayYMaximum=4.2312214706255107  DataLoggingVariableName=ScopeData50
  Scope4 : Scope  Commented=on
      settings: DataLoggingVariableName=ScopeData_rdotSmc
  Subtract : Sum  Inputs=+-
  Sum3 : Sum  Inputs=|++
  Sum4 : Sum  Inputs=|+-
  xi1 : Gain  Gain=xi
  r_dotSmc : Outport
  tag scope: r_dotSmc=global
  wires:
  Sum4/1 -> xi1/1
  xi1/1 -> Scope1/2, Subtract/2
  Discrete Derivative1/1 -> Sum4/1
  Sum3/1 -> Scope1/1, Subtract/1
  Discrete Derivative/1 -> Sum3/2
  s_dot/1 -> Sum3/1
  Discrete Derivative2/1 -> Sum4/2
  Subtract/1 -> Scope4/1, [r_dotSmc], Scope3/1, Scope2/1, Median Filter/1  "r_dotSmc"
  Median Filter/1 -> r_dotSmc/1, Scope/1, Scope3/2  "r_dotSmc"
  r_des/1 -> Discrete Derivative/1
  beta/1 -> Discrete Derivative1/1
  beta_des/1 -> Discrete Derivative2/1

== system SDV_HIL/HIL/UDP Transmit PC -> VCU/Subsystem/Torque Vectoring/Upper-Level Control/s Calculation ==
  r_des : Inport
  beta_des : Inport  Port=2
  r : Inport  Port=3
  beta : Inport  Port=4
  Add : Sum
  Mux : Mux  Inputs=2
  Mux1 : Mux  Inputs=2
  Mux2 : Mux  Inputs=2
  Radians to Degrees : simulink_extras/Transformations/Radians to Degrees
  Radians to Degrees1 : simulink_extras/Transformations/Radians to Degrees
  Scope : Scope  Commented=on  NumInputPorts=2
      settings: ActiveDisplayYMinimum=-0.28171028288036076  ActiveDisplayYMaximum=0.28186498160357804  DataLoggingVariableName=ScopeData27
  Scope1 : Scope  Commented=on  NumInputPorts=2
      settings: ActiveDisplayYMinimum=-0.14632790991396921  ActiveDisplayYMaximum=0.14632790991396921  DataLoggingVariableName=ScopeData28
  Scope2 : Scope  Commented=on
      settings: ActiveDisplayYMinimum=-15.502678068808111  ActiveDisplayYMaximum=19.821343432137777  DataLoggingVariableName=ScopeData_rRespons
  Scope3 : Scope  Commented=on
      settings: ActiveDisplayYMinimum=-5.2852193383146249  ActiveDisplayYMaximum=3.969293753648568  DataLoggingVariableName=ScopeData_betaRespons
  Sum1 : Sum  Inputs=|+-
  Sum2 : Sum  Inputs=|+-
  xi : Gain  Gain=xi
  s : Outport
  tag scope: rBeta_respons=global
  wires:
  Add/1 -> s/1
  xi/1 -> Add/2
  Sum2/1 -> xi/1  "err_beta"
  Sum1/1 -> Add/1  "error_yawrate"
  r/1 -> Mux/2, Scope/2, Sum1/1
  r_des/1 -> Mux/1, Scope/1, Sum1/2
  beta/1 -> Mux1/2, Scope1/2, Sum2/1
  Mux/1 -> Mux2/1, Radians to Degrees/1
  Mux1/1 -> Mux2/2, Radians to Degrees1/1
  Mux2/1 -> [rBeta_respons]
  Radians to Degrees/1 -> Scope2/1
  Radians to Degrees1/1 -> Scope3/1
  beta_des/1 -> Mux1/1, Scope1/1, Sum2/2

== system SDV_HIL/Draft1/UDP Transmit PC -> VCU1/Subsystem/4 Wheel Steering system/Kinematik/YO equation/Subsystem ==
  In2 : Inport
  In4 : Inport  Port=2
  Abs1 : Abs  SaturateOnIntegerOverflow=off
  Add1 : Sum
  Atan2 : Trigonometry  Operator=tan
  Constant1 : Constant  Value=0
  Deg2Rad1 : Gain  Gain=3.14/180
  Display2 : Display
  Display3 : Display
  Divide1 : Product  Inputs=*/
  Gain2 : Gain  Gain=1/2
  Gain3 : Gain  Gain=-1
  Switch2 : Switch  Criteria=u2 ~= 0  SaturateOnIntegerOverflow=off  InputSameDT=off
  Switch3 : Switch  Criteria=u2 > Threshold  SaturateOnIntegerOverflow=off  InputSameDT=off
  "WheelBase, m1" : Constant  Value=3.100
  YO = R2 : Display
  R2 : Outport
  YO1 : Outport  Port=2
  wires:
  In2/1 -> Add1/1
  In4/1 -> Abs1/1, Switch2/2, Switch3/2
  Constant1/1 -> Switch2/3
  Atan2/1 -> Switch2/1
  Deg2Rad1/1 -> Atan2/1
  Divide1/1 -> Add1/2
  Gain2/1 -> Divide1/1, Display3/1
  Switch2/1 -> Display2/1, Divide1/2
  Switch3/1 -> YO1/1
  Add1/1 -> R2/1, YO = R2/1, Gain3/1, Switch3/1
  Abs1/1 -> Deg2Rad1/1
  "WheelBase, m1"/1 -> Gain2/1
  Gain3/1 -> Switch3/3

== system SDV_HIL/Draft1/UDP Transmit PC -> VCU1/Subsystem/Torque Vectoring/Upper-Level Control/r_dot Calculation/Draft ==
  Discrete Transfer Fcn1 : DiscreteTransferFcn  LoadFcn=dspblkCoreblockFVToolHelper(gcbh,'load');  Numerator="[0.000944691843840\t0.001889383687680\t0.000944691843840]"  Denominator="[1.000000000000000\t-1.911197067426073\t0.914975834801434]"
      settings: CopyFcn=dspblkCoreblockFVToolHelper(gcbh,'copy');  DeleteFcn=dspblkCoreblockFVToolHelper(gcbh,'close');  ModelCloseFcn=dspblkCoreblockFVToolHelper(gcbh,'close');  PreSaveFcn=dspblkCoreblockFVToolHelper(gcbh,'presave');  PostSaveFcn=dspblkCoreblockFVToolHelper(gcbh,'postsave');  CloseFcn=dspblkCoreblockFVToolHelper(gcbh,'close');
  Rate Limiter : RateLimiter  RisingSlewLimit=35  FallingSlewLimit=-35  SampleTimeMode=inherited
  Scope2 : Scope  NumInputPorts=2
      settings: ActiveDisplayYMinimum=2.8695401701631194  ActiveDisplayYMaximum=2.8931693462345129  DataLoggingVariableName=ScopeData20
  Scope5 : Scope  NumInputPorts=2
      settings: ActiveDisplayYMinimum=-10.107684663391382  ActiveDisplayYMaximum=10.708654843908857  DataLoggingVariableName=ScopeData20
  wires:
  Rate Limiter/1 -> Scope2/2
  Discrete Transfer Fcn1/1 -> Scope5/2

== system SDV_HIL/HIL/UDP Transmit PC -> VCU/Subsystem/4 Wheel Steering system/Kinematik/YO equation/Subsystem ==
  In2 : Inport
  In4 : Inport  Port=2
  Abs1 : Abs  SaturateOnIntegerOverflow=off
  Add1 : Sum
  Atan2 : Trigonometry  Operator=tan
  Constant1 : Constant  Value=0
  Deg2Rad1 : Gain  Gain=3.14/180
  Display2 : Display
  Display3 : Display
  Divide1 : Product  Inputs=*/
  Gain2 : Gain  Gain=1/2
  Gain3 : Gain  Gain=-1
  Switch2 : Switch  Criteria=u2 ~= 0  SaturateOnIntegerOverflow=off  InputSameDT=off
  Switch3 : Switch  Criteria=u2 > Threshold  SaturateOnIntegerOverflow=off  InputSameDT=off
  "WheelBase, m1" : Constant  Value=3.100
  YO = R2 : Display
  R2 : Outport
  YO1 : Outport  Port=2
  wires:
  In2/1 -> Add1/1
  In4/1 -> Abs1/1, Switch2/2, Switch3/2
  Constant1/1 -> Switch2/3
  Atan2/1 -> Switch2/1
  Deg2Rad1/1 -> Atan2/1
  Divide1/1 -> Add1/2
  Gain2/1 -> Divide1/1, Display3/1
  Switch2/1 -> Display2/1, Divide1/2
  Switch3/1 -> YO1/1
  Add1/1 -> R2/1, YO = R2/1, Gain3/1, Switch3/1
  Abs1/1 -> Deg2Rad1/1
  "WheelBase, m1"/1 -> Gain2/1
  Gain3/1 -> Switch3/3

== system SDV_HIL/HIL/UDP Transmit PC -> VCU/Subsystem/Torque Vectoring/Upper-Level Control/r_dot Calculation/Draft ==
  Discrete Transfer Fcn1 : DiscreteTransferFcn  LoadFcn=dspblkCoreblockFVToolHelper(gcbh,'load');  Numerator="[0.000944691843840\t0.001889383687680\t0.000944691843840]"  Denominator="[1.000000000000000\t-1.911197067426073\t0.914975834801434]"
      settings: CopyFcn=dspblkCoreblockFVToolHelper(gcbh,'copy');  DeleteFcn=dspblkCoreblockFVToolHelper(gcbh,'close');  ModelCloseFcn=dspblkCoreblockFVToolHelper(gcbh,'close');  PreSaveFcn=dspblkCoreblockFVToolHelper(gcbh,'presave');  PostSaveFcn=dspblkCoreblockFVToolHelper(gcbh,'postsave');  CloseFcn=dspblkCoreblockFVToolHelper(gcbh,'close');
  Rate Limiter : RateLimiter  RisingSlewLimit=35  FallingSlewLimit=-35  SampleTimeMode=inherited
  Scope2 : Scope  NumInputPorts=2
      settings: ActiveDisplayYMinimum=2.8695401701631194  ActiveDisplayYMaximum=2.8931693462345129  DataLoggingVariableName=ScopeData20
  Scope5 : Scope  NumInputPorts=2
      settings: ActiveDisplayYMinimum=-10.107684663391382  ActiveDisplayYMaximum=10.708654843908857  DataLoggingVariableName=ScopeData20
  wires:
  Rate Limiter/1 -> Scope2/2
  Discrete Transfer Fcn1/1 -> Scope5/2

== matlab function SDV_HIL/HIL/UDP Transmit PC -> VCU/Subsystem/4 Wheel Steering system/Kinematik/YO equation/MATLAB Function ==
  data: Steer input; R1 output; Y0 output
function [R1,Y0] = fcn(Steer)

Hwb = 3.1/2;
Hwt = 1.49/2;
Y0 = 0;
R1 = 0;

k = tan(deg2rad(abs(Steer)));

if Steer == 0
    n = 0;
else
    n = k;
end

R1 = (Hwb/n)+Hwt;

if Steer > 0
    Y0 = R1;
elseif Steer < 0
    Y0 = R1*(-1);
else
    Y0 = 0;
end

== matlab function SDV_HIL/HIL/UDP Receive ZCU -> PC/MATLAB Function ==
  data: payload input; FL output; FR output; RL output; RR output; seqRecv output
function [FL, FR, RL, RR, seqRecv] = recvZCUFrame(payload)

% -------------------------------------------------------------------------
% recvZCUFrame
% Receive UDP frame from ZCU and decode per-wheel data
%
% Frame format (7 bytes):
% [1] Header = 0xCA
% [2] ID     = 1..4
% [3:4] Speed (int16)
% [5:6] Angle (int16)
% [7] Seq    (uint8)
% -------------------------------------------------------------------------

% =======================
% Persistent storage

persistent data
if isempty(data)
    % data(row,:) = [angle speed seq]
    data = zeros(4,3,'double');
end

% =======================
% Process incoming payload

data = processOne(payload, data);

% =======================
% Outputs

FL = data(1,1:2);
FR = data(2,1:2);
RL = data(3,1:2);
RR = data(4,1:2);

seqRecv = data(:,3);

% =======================
% Nested function

    function dataOut = processOne(payloadIn, dataIn)

        dataOut = dataIn;

        % Length check
        if numel(payloadIn) < 7
            return;
        end

        % Header check
        if payloadIn(1) ~= uint8(hex2dec('CB'))
            return;
        end

        % ID check
        id = payloadIn(2);
        if id < 1 || id > 4
            return;
        end

        % Decode
        speed = double(typecast(uint8(payloadIn(3:4)), 'int16'));
        angle = double(typecast(uint8(payloadIn(5:6)), 'int16'));
        seq   = double(payloadIn(7));

        dataOut(id,1) = speed;
        dataOut(id,2) = angle;
        dataOut(id,3) = seq;
    end
end

== matlab function SDV_HIL/HIL/Driver/Logitech G29/MATLAB Function ==
  data: btn input; state output
function state = fnc(btn)
%#codegen
% Start/Stop toggle dari 1 tombol joystick
% btn  : input tombol (0 atau 1, tipe double)
% state: output status (0=stop, 1=start)

persistent s last
if isempty(s)
    s = 0;      % status awal stop
    last = 0;   % tombol sebelumnya
end

% pastikan semua double
btn  = double(btn);
s    = double(s);
last = double(last);

% deteksi rising edge
if (btn == 1) && (last == 0)
    s = 1 - s;  % toggle
end

% simpan status tombol sebelumnya
last = btn;

% keluaran status
state = s;
end

== matlab function SDV_HIL/HIL/UDP Transmit PC -> VCU/Subsystem/Torque Vectoring/Speed Control/MATLAB Function ==
  data: Fx_total input; y output; Vx_des input; Vx input
function y = fcn(Fx_total, Vx_des, Vx)

if Vx_des > 1
    y = Fx_total;    
else
    y = 0;
end

== matlab function SDV_HIL/Draft1/Driver Logi G1/MATLAB Function ==
  data: btn input; state output
function state = fnc(btn)
%#codegen
% Start/Stop toggle dari 1 tombol joystick
% btn  : input tombol (0 atau 1, tipe double)
% state: output status (0=stop, 1=start)

persistent s last
if isempty(s)
    s = 0;      % status awal stop
    last = 0;   % tombol sebelumnya
end

% pastikan semua double
btn  = double(btn);
s    = double(s);
last = double(last);

% deteksi rising edge
if (btn == 1) && (last == 0)
    s = 1 - s;  % toggle
end

% simpan status tombol sebelumnya
last = btn;

% keluaran status
state = s;
end
